simulink model "GaitAlgorithm_arduino_V5_2024b"  (R2024b)
settings: Solver=FixedStepAuto  StartTime=0.0  StopTime=inf  RelTol=1e-3  EnableMultiTasking=on
undefined symbols (not defined in the file): f
libraries: simulink x16, mcp2515lib x13, eeGeneralControl x4, arduinolib x2, instrumentlib x2, arduinosensorlib x2
(part 2 of 2)

== system GaitAlgorithm_arduino_V5_2024b/CANbegin/setup/setCANspeed/mcp2515_writeRegister1 ==
  In : Inport
  address : Inport  Port=2  OutDataTypeStr=uint8
  value : Inport  Port=3  OutDataTypeStr=uint8
  MCP_WRITE : Constant  Value=2  OutDataTypeStr=uint8
  SPI driver : mcp2515lib/CAN application/mcp2515 driver/SPI driver  SystemSampleTime=-1  VariantActivationTime=update diagram  AllowFlexibleInterface=on  Latency=0  AutoFrameSizeCalculation=off
      settings: SourceProductName=CAN device driver for mcp2515
  Selector : Selector  IndexMode=Zero-based  InputPortWidth=3  IndexOptions=Index vector (dialog)  Indices=0  OutputSizes=1
  Temporary buffer : DataStoreWrite  DataStoreName=temp_1byte  IndexOptions=Index vector (dialog)  Indices=1  OutputSizes=1
  Vector Concatenate : Concatenate  NumInputs=3
  Out : Outport
  wires:
  SPI driver/1 -> Selector/1
  Selector/1 -> Temporary buffer/1
  In/1 -> Out/1
  Vector Concatenate/1 -> SPI driver/1
  value/1 -> Vector Concatenate/3
  address/1 -> Vector Concatenate/2
  MCP_WRITE/1 -> Vector Concatenate/1

== system GaitAlgorithm_arduino_V5_2024b/CANbegin/setup/setCANspeed/mcp2515_writeRegister2 ==
  In : Inport
  address : Inport  Port=2  OutDataTypeStr=uint8
  value : Inport  Port=3  OutDataTypeStr=uint8
  MCP_WRITE : Constant  Value=2  OutDataTypeStr=uint8
  SPI driver : mcp2515lib/CAN application/mcp2515 driver/SPI driver  SystemSampleTime=-1  VariantActivationTime=update diagram  AllowFlexibleInterface=on  Latency=0  AutoFrameSizeCalculation=off
      settings: SourceProductName=CAN device driver for mcp2515
  Selector : Selector  IndexMode=Zero-based  InputPortWidth=3  IndexOptions=Index vector (dialog)  Indices=0  OutputSizes=1
  Temporary buffer : DataStoreWrite  DataStoreName=temp_1byte  IndexOptions=Index vector (dialog)  Indices=1  OutputSizes=1
  Vector Concatenate : Concatenate  NumInputs=3
  Out : Outport
  wires:
  SPI driver/1 -> Selector/1
  Selector/1 -> Temporary buffer/1
  In/1 -> Out/1
  Vector Concatenate/1 -> SPI driver/1
  value/1 -> Vector Concatenate/3
  address/1 -> Vector Concatenate/2
  MCP_WRITE/1 -> Vector Concatenate/1

== system GaitAlgorithm_arduino_V5_2024b/CANbegin/setup/setCANspeed/mcp2515_writeRegister3 ==
  In : Inport
  address : Inport  Port=2  OutDataTypeStr=uint8
  value : Inport  Port=3  OutDataTypeStr=uint8
  MCP_WRITE : Constant  Value=2  OutDataTypeStr=uint8
  SPI driver : mcp2515lib/CAN application/mcp2515 driver/SPI driver  SystemSampleTime=-1  VariantActivationTime=update diagram  AllowFlexibleInterface=on  Latency=0  AutoFrameSizeCalculation=off
      settings: SourceProductName=CAN device driver for mcp2515
  Selector : Selector  IndexMode=Zero-based  InputPortWidth=3  IndexOptions=Index vector (dialog)  Indices=0  OutputSizes=1
  Temporary buffer : DataStoreWrite  DataStoreName=temp_1byte  IndexOptions=Index vector (dialog)  Indices=1  OutputSizes=1
  Vector Concatenate : Concatenate  NumInputs=3
  Out : Outport
  wires:
  SPI driver/1 -> Selector/1
  Selector/1 -> Temporary buffer/1
  In/1 -> Out/1
  Vector Concatenate/1 -> SPI driver/1
  value/1 -> Vector Concatenate/3
  address/1 -> Vector Concatenate/2
  MCP_WRITE/1 -> Vector Concatenate/1

== system GaitAlgorithm_arduino_V5_2024b/CANreceive/readRxBuffer/getID/checkExtendedId ==
  SIDL : Inport
  Bitmask_EXIDE : simulink/Logic and Bit Operations/Bitwise Operator  logicop=AND  UseBitMask=on  BitMask=bin2dec('00001000')  BitMaskRealWorld=Stored Integer
  MCP_TXB_EXIDE_M : Constant  Value=hex2dec('08')  OutDataTypeStr=uint8
  Relational Operator : RelationalOperator  Operator===  OutDataTypeStr=boolean  InputSameDT=off
  ext : Outport
  wires:
  Relational Operator/1 -> ext/1
  MCP_TXB_EXIDE_M/1 -> Relational Operator/1
  Bitmask_EXIDE/1 -> Relational Operator/2
  SIDL/1 -> Bitmask_EXIDE/1

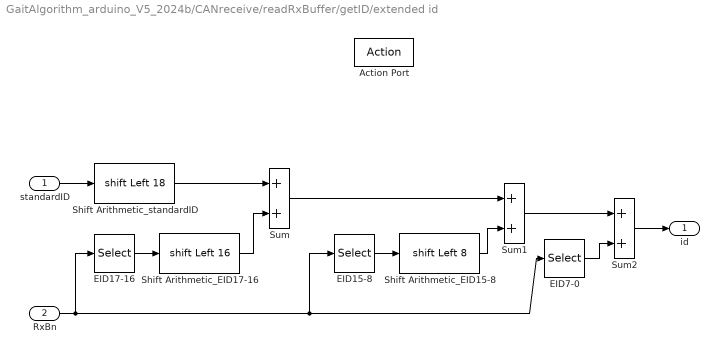
== system GaitAlgorithm_arduino_V5_2024b/CANreceive/readRxBuffer/getID/extended id ==
  standardID : Inport
  RxBn : Inport  Port=2
  Action Port : ActionPort  ActionPortLabel=if(u1 == 1)
  EID15-8 : Selector  IndexMode=Zero-based  InputPortWidth=13  IndexOptions=Index vector (dialog)  Indices=2  OutputSizes=1
  EID17-16 : Selector  IndexMode=Zero-based  InputPortWidth=13  IndexOptions=Index vector (dialog)  Indices=1  OutputSizes=1
  EID7-0 : Selector  IndexMode=Zero-based  InputPortWidth=13  IndexOptions=Index vector (dialog)  Indices=3  OutputSizes=1
  Shift Arithmetic_EID15-8 : ArithShift  BitShiftNumber=8  BitShiftDirection=Left
  Shift Arithmetic_EID17-16 : ArithShift  BitShiftNumber=16  BitShiftDirection=Left
  Shift Arithmetic_standardID : ArithShift  BitShiftNumber=18  BitShiftDirection=Left
  Sum : Sum
  Sum1 : Sum
  Sum2 : Sum
  id : Outport
  wires:
  Sum2/1 -> id/1
  standardID/1 -> Shift Arithmetic_standardID/1
  Shift Arithmetic_standardID/1 -> Sum/1
  EID17-16/1 -> Shift Arithmetic_EID17-16/1
  Shift Arithmetic_EID17-16/1 -> Sum/2
  Sum/1 -> Sum1/1
  Shift Arithmetic_EID15-8/1 -> Sum1/2
  EID15-8/1 -> Shift Arithmetic_EID15-8/1
  Sum1/1 -> Sum2/1
  RxBn/1 -> EID7-0/1, EID15-8/1, EID17-16/1
  EID7-0/1 -> Sum2/2

== system GaitAlgorithm_arduino_V5_2024b/CANreceive/readRxBuffer/getID/getStandardID ==
  SIDL : Inport
  SIDH : Inport  Port=2
  Bitmask_SID2-0 : simulink/Logic and Bit Operations/Bitwise Operator  logicop=AND  UseBitMask=on  BitMask=bin2dec('11100000')  BitMaskRealWorld=Stored Integer
  Data Type Conversion : DataTypeConversion  OutDataTypeStr=uint32  SaturateOnIntegerOverflow=off  RndMeth=Floor
  Shift Arithmetic_SID10-3 : ArithShift  BitShiftNumber=3  BitShiftDirection=Left
  Shift Arithmetic_SID2-0 : ArithShift  BitShiftNumber=5  BitShiftDirection=Right
  Sum1 : Sum
  stadardID : Outport
  wires:
  Sum1/1 -> stadardID/1
  Shift Arithmetic_SID2-0/1 -> Sum1/1
  Shift Arithmetic_SID10-3/1 -> Sum1/2
  SIDL/1 -> Bitmask_SID2-0/1
  SIDH/1 -> Data Type Conversion/1
  Bitmask_SID2-0/1 -> Shift Arithmetic_SID2-0/1
  Data Type Conversion/1 -> Shift Arithmetic_SID10-3/1

== system GaitAlgorithm_arduino_V5_2024b/CANreceive/readRxBuffer/getID/standard id ==
  stadardID : Inport
  Action Port : ActionPort  ActionPortLabel=else
  id : Outport
  wires:
  stadardID/1 -> id/1

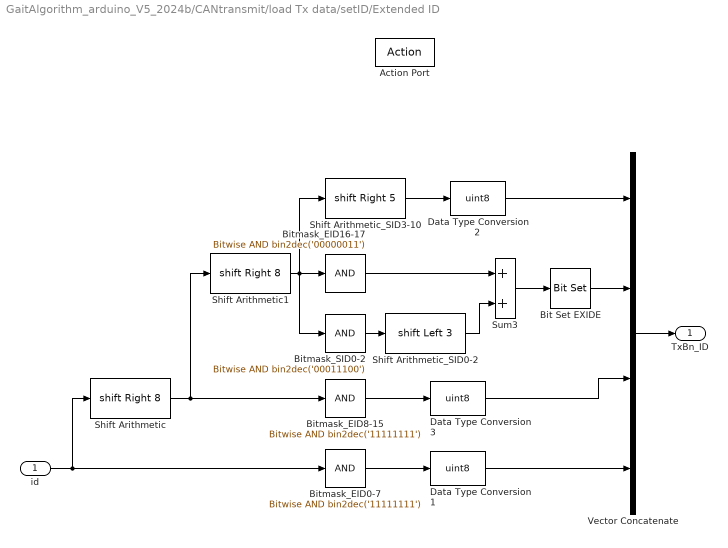
== system GaitAlgorithm_arduino_V5_2024b/CANtransmit/load Tx data/setID/Extended ID ==
  id : Inport
  Action Port : ActionPort  ActionPortLabel=if(u1 > 0)
  Bit Set EXIDE : simulink/Logic and Bit Operations/Bit Set  iBit=3
  Bitmask_EID0-7 : simulink/Logic and Bit Operations/Bitwise Operator  logicop=AND  UseBitMask=on  BitMask=bin2dec('11111111')  BitMaskRealWorld=Stored Integer
  Bitmask_EID16-17 : simulink/Logic and Bit Operations/Bitwise Operator  logicop=AND  UseBitMask=on  BitMask=bin2dec('00000011')  BitMaskRealWorld=Stored Integer
  Bitmask_EID8-15 : simulink/Logic and Bit Operations/Bitwise Operator  logicop=AND  UseBitMask=on  BitMask=bin2dec('11111111')  BitMaskRealWorld=Stored Integer
  Bitmask_SID0-2 : simulink/Logic and Bit Operations/Bitwise Operator  logicop=AND  UseBitMask=on  BitMask=bin2dec('00011100')  BitMaskRealWorld=Stored Integer
  Data Type Conversion1 : DataTypeConversion  OutDataTypeStr=uint8  RndMeth=Simplest  SaturateOnIntegerOverflow=off
  Data Type Conversion2 : DataTypeConversion  OutDataTypeStr=uint8  RndMeth=Simplest  SaturateOnIntegerOverflow=off
  Data Type Conversion3 : DataTypeConversion  OutDataTypeStr=uint8  RndMeth=Simplest  SaturateOnIntegerOverflow=off
  Shift Arithmetic : ArithShift  BitShiftNumber=8  BitShiftDirection=Right
  Shift Arithmetic1 : ArithShift  BitShiftNumber=8  BitShiftDirection=Right
  Shift Arithmetic_SID0-2 : ArithShift  BitShiftNumber=3  BitShiftDirection=Left
  Shift Arithmetic_SID3-10 : ArithShift  BitShiftNumber=5  BitShiftDirection=Right
  Sum3 : Sum  OutDataTypeStr=uint8
  Vector Concatenate : Concatenate  NumInputs=4
  TxBn_ID : Outport
  wires:
  Vector Concatenate/1 -> TxBn_ID/1
  id/1 -> Shift Arithmetic/1, Bitmask_EID0-7/1
  Bitmask_EID0-7/1 -> Data Type Conversion1/1
  Data Type Conversion1/1 -> Vector Concatenate/4
  Shift Arithmetic/1 -> Shift Arithmetic1/1, Bitmask_EID8-15/1
  Bitmask_EID8-15/1 -> Data Type Conversion3/1
  Data Type Conversion3/1 -> Vector Concatenate/3
  Shift Arithmetic1/1 -> Shift Arithmetic_SID3-10/1, Bitmask_SID0-2/1, Bitmask_EID16-17/1
  Sum3/1 -> Bit Set EXIDE/1
  Bitmask_EID16-17/1 -> Sum3/1
  Bitmask_SID0-2/1 -> Shift Arithmetic_SID0-2/1
  Shift Arithmetic_SID0-2/1 -> Sum3/2
  Bit Set EXIDE/1 -> Vector Concatenate/2
  Shift Arithmetic_SID3-10/1 -> Data Type Conversion2/1
  Data Type Conversion2/1 -> Vector Concatenate/1

== system GaitAlgorithm_arduino_V5_2024b/CANtransmit/load Tx data/setID/Standard ID ==
  id : Inport
  Action Port : ActionPort  ActionPortLabel=else
  Vector Concatenate : Concatenate  NumInputs=4
  convert_ID : Subsystem  TreatAsAtomicUnit=on
  no data : Constant  Value=0  OutDataTypeStr=uint8
  TxBn_ID : Outport
  wires:
  Vector Concatenate/1 -> TxBn_ID/1
  no data/1 -> Vector Concatenate/3, Vector Concatenate/4
  convert_ID/2(SIDL) -> Vector Concatenate/2
  id/1 -> convert_ID/1(id)
  convert_ID/1(SIDH) -> Vector Concatenate/1

== system GaitAlgorithm_arduino_V5_2024b/CANtransmit/load Tx data/setID/Standard ID/convert_ID ==
  id : Inport
  Bitmask_SID0-10 : simulink/Logic and Bit Operations/Bitwise Operator  logicop=AND  UseBitMask=on  BitMask=bin2dec('0000011111111111')  BitMaskRealWorld=Stored Integer
  Bitmask_SID0-2 : simulink/Logic and Bit Operations/Bitwise Operator  logicop=AND  UseBitMask=on  BitMask=bin2dec('0000000011100000')  BitMaskRealWorld=Stored Integer
  Data Type Conversion1 : DataTypeConversion  OutDataTypeStr=uint8  RndMeth=Simplest  SaturateOnIntegerOverflow=off
  Data Type Conversion2 : DataTypeConversion  OutDataTypeStr=uint8  RndMeth=Simplest  SaturateOnIntegerOverflow=off
  Shift Arithmetic1 : ArithShift  BitShiftNumber=3  BitShiftDirection=Right
  Shift Arithmetic2 : ArithShift  BitShiftNumber=5  BitShiftDirection=Left
  SIDH : Outport
  SIDL : Outport  Port=2
  wires:
  Shift Arithmetic1/1 -> Data Type Conversion1/1
  Data Type Conversion1/1 -> SIDH/1
  Bitmask_SID0-10/1 -> Shift Arithmetic2/1, Shift Arithmetic1/1
  Data Type Conversion2/1 -> SIDL/1
  Shift Arithmetic2/1 -> Bitmask_SID0-2/1
  id/1 -> Bitmask_SID0-10/1
  Bitmask_SID0-2/1 -> Data Type Conversion2/1

== matlab function GaitAlgorithm_arduino_V5_2024b/Enabled Subsystem1/MATLAB Function ==
  data: angle_deg input; canBytes output
function canBytes = angle2CANByte(angle_deg)
    % 출력 canBytes 속성 명시
    canBytes = uint8(zeros(1,4)); 
    
    % 1. 각도를 int32로 변환 (0.0001° 단위)
    pos_int32 = int32(round(angle_deg * 10000));
    
    % 2. 4바이트 리틀 엔디안 변환
    canBytes = typecast(pos_int32, 'uint8');  % [1x4]
   
end

== matlab function GaitAlgorithm_arduino_V5_2024b/Enabled Subsystem4/MATLAB Function1 ==
  data: angle_deg input; canBytes output
function canBytes = angle2CANByte(angle_deg)
    % 출력 canBytes 속성 명시
    Bytes = uint8(zeros(1,4));
    canBytes = uint8(zeros(1,4));
    
    % 1. 각도를 int32로 변환 (0.0001° 단위)
    pos_int32= int32(round(angle_deg * 10000));
    
    % 2. 4바이트 리틀 엔디안 변환
    Bytes = typecast(pos_int32, 'uint8');  % [1x4]

        % 3. 바이트 순서 뒤집기 → Big Endian
    canBytes = Bytes(end:-1:1);  % MSB 먼저
   
end

== matlab function GaitAlgorithm_arduino_V5_2024b/Enabled Subsystem3/MATLAB Function1 ==
  data: angle_deg input; canBytes output
function canBytes = angle2CANByte(angle_deg)
    % 출력 canBytes 속성 명시
    Bytes = uint8(zeros(1,4));
    canBytes = uint8(zeros(1,4));
    
    % 1. 각도를 int32로 변환 (0.0001° 단위)
    pos_int32= int32(round(angle_deg * 10000));
    
    % 2. 4바이트 리틀 엔디안 변환
    Bytes = typecast(pos_int32, 'uint8');  % [1x4]

        % 3. 바이트 순서 뒤집기 → Big Endian
    canBytes = Bytes(end:-1:1);  % MSB 먼저
   
end

== matlab function GaitAlgorithm_arduino_V5_2024b/Enabled Subsystem1/MATLAB Function1 ==
  data: angle_deg input; canBytes output
function canBytes = angle2CANByte(angle_deg)
    % 출력 canBytes 속성 명시
    Bytes = uint8(zeros(1,4));
    canBytes = uint8(zeros(1,4));
    
    % 1. 각도를 int32로 변환 (0.0001° 단위)
    pos_int32= int32(round(angle_deg * 10000));
    
    % 2. 4바이트 리틀 엔디안 변환
    Bytes = typecast(pos_int32, 'uint8');  % [1x4]

        % 3. 바이트 순서 뒤집기 → Big Endian
    canBytes = Bytes(end:-1:1);  % MSB 먼저
   
end
